simulink model "PID"  (R2019a)
settings: Solver=FixedStepDiscrete  StartTime=0.0  StopTime=10.0  RelTol=1e-3
settings Model: Creator=yuzehong  LastModifiedBy=mluser
settings OptimizationCC: DefaultParameterBehavior=Inlined  UseDivisionForNetSlopeComputation=on  GainParamInheritBuiltInType=on  UseFloatMulNetSlope=on  InlineInvariantSignals=on  OptimizeBlockIOStorage=off  BufferReuse=off  GlobalBufferReuse=off  ExpressionFolding=off  EnableMemcpy=off  PassReuseOutputArgsAs=Individual arguments  LocalBlockOutputs=off  ZeroExternalMemoryAtStartup=off  ZeroInternalMemoryAtStartup=off  NoFixptDivByZeroProtection=on  EfficientFloat2IntCast=on  LifeSpan=1  OptimizeDataStoreBuffers=off  BusAssignmentInplaceUpdate=off  OptimizationLevel=level0  OptimizationPriority=Speed  MultiThreadedLoops=on
settings DebuggingCC: ParameterTunabilityLossMsg=error  SFMachineParentedDataDiag=error
settings HardwareCC: ProdBitPerLong=64  ProdHWDeviceType=Intel->x86-64 (Linux 64)
settings SFSimCC: MATLABDynamicMemAlloc=off
settings RTWCC: SystemTargetFile=ert.tlc  GenCodeOnly=on  TemplateMakefile=ert_default_tmf
settings CodeAppCC: GenerateComments=off  IgnoreCustomStorageClasses=off  OperatorAnnotations=on  SimulinkDataObjDesc=on  SFDataObjDesc=on  CustomSymbolStrGlobalVar=rt$N$M  CustomSymbolStrType=$N$M  CustomSymbolStrFcn=$N$M$F  CustomSymbolStrMacro=$N$M  SimulinkBlockComments=off
settings ERTTargetCC: TargetLangStandard=C99 (ISO)  CodeReplacementLibrary=Intel AVX (Linux)  GenerateSampleERTMain=on  IncludeMdlTerminateFcn=off  CombineSignalStateStructs=on  SuppressErrorStatus=on  SupportAbsoluteTime=off  SupportNonFinite=off  SupportComplex=off  InlinedParameterPlacement=NonHierarchical  ERTCustomFileTemplate=example_file_process.tlc  ERTFilePackagingFormat=CompactWithDataFile

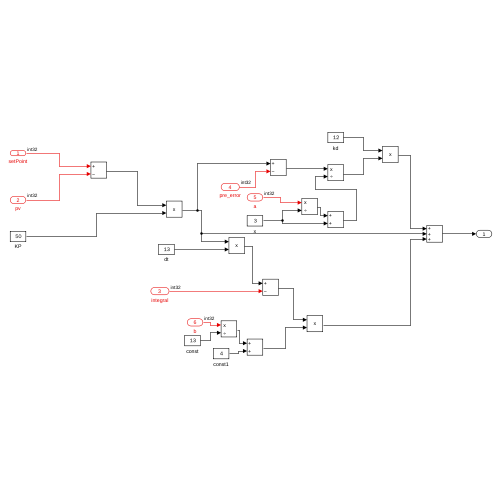
[thumbnail: Simulink's stored preview of the top-level diagram]
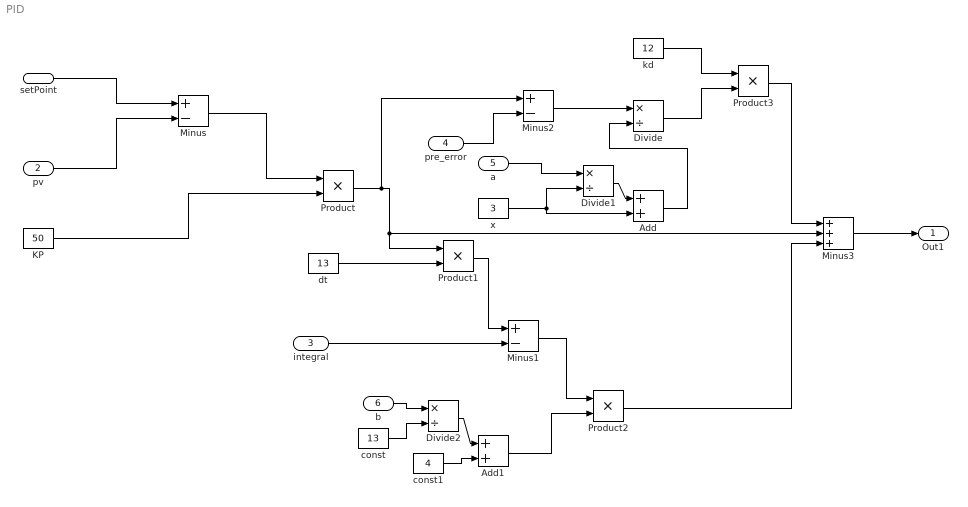
== system PID ==
  setPoint : Inport  OutDataTypeStr=int32  PortDimensions=1
  pv : Inport  Port=2  OutDataTypeStr=int32  PortDimensions=1
  integral : Inport  Port=3  OutDataTypeStr=int32  PortDimensions=1
  pre_error : Inport  Port=4  OutDataTypeStr=int32  PortDimensions=1
  a : Inport  Port=5  OutDataTypeStr=int32  PortDimensions=1
  b : Inport  Port=6  OutDataTypeStr=int32  PortDimensions=1
  Add : Sum  AccumDataTypeStr=int32  OutDataTypeStr=int32
  Add1 : Sum  AccumDataTypeStr=int32  OutDataTypeStr=int32
  Divide : Product  Inputs=*/  OutDataTypeStr=int32  RndMeth=Simplest
  Divide1 : Product  Inputs=*/  OutDataTypeStr=int32  RndMeth=Simplest
  Divide2 : Product  Inputs=*/  OutDataTypeStr=int32  RndMeth=Simplest
  KP : Constant  Value=50  OutDataTypeStr=int32
  Minus : Sum  Inputs=+-  OutDataTypeStr=int32
  Minus1 : Sum  Inputs=+-  AccumDataTypeStr=int32  OutDataTypeStr=int32
  Minus2 : Sum  Inputs=+-  AccumDataTypeStr=int32
  Minus3 : Sum  Inputs=+++  OutDataTypeStr=int32
  Product{,1..3} (4 alike) : Product  OutDataTypeStr=int32
  const : Constant  Value=13  OutDataTypeStr=int32
  const1 : Constant  Value=4  OutDataTypeStr=int32
  dt : Constant  Value=13  OutDataTypeStr=int32
  kd : Constant  Value=12  OutDataTypeStr=int32
  x : Constant  Value=3  OutDataTypeStr=int32
  Out1 : Outport
  wires:
  setPoint/1 -> Minus/1
  pv/1 -> Minus/2
  Minus/1 -> Product/1
  KP/1 -> Product/2
  Product/1 -> Minus3/2, Product1/1, Minus2/1
  dt/1 -> Product1/2
  integral/1 -> Minus1/2
  Product1/1 -> Minus1/1
  Minus1/1 -> Product2/1
  pre_error/1 -> Minus2/2
  Minus2/1 -> Divide/1
  kd/1 -> Product3/1
  Divide/1 -> Product3/2
  Product3/1 -> Minus3/1
  Product2/1 -> Minus3/3
  Minus3/1 -> Out1/1
  a/1 -> Divide1/1
  x/1 -> Divide1/2, Add/2
  Divide1/1 -> Add/1
  Add/1 -> Divide/2
  b/1 -> Divide2/1
  const/1 -> Divide2/2
  Divide2/1 -> Add1/1
  const1/1 -> Add1/2
  Add1/1 -> Product2/2
